simulink library "COMH"  (R2016b)
settings: Solver=ode45  StartTime=0.0  StopTime=10.0  RelTol=1e-3  EnableMultiTasking=on
undefined symbols (not defined in the file): CAL_EncoderSampleTime, CAL_FilterResetThd, CAL_fullCircle_DEG, CAL_MeasureNoise, CAL_NORTH, CAL_ProcessNoise, CAL_ROB_ERRVAL, CAL_ROBO_LENG_mm, CAL_thetaGain, CONST_ONE_UINT16, CONST_ZERO_UINT16, CONST_ZeroDeg, ENU_ROB_NONE
libraries: ThetaOverFlowFilter x1, movingAverage_1ms_to_5ms x1
settings Model: Creator=oelkawok  LastModifiedBy=oelkawok
settings DataIOCC: LimitDataPoints=on
settings OptimizationCC: LifeSpan=inf
settings DebuggingCC: AllowSymbolicDim=off  SFUnexpectedBacktrackingDiag=warning  SFNoUnconditionalDefaultTransitionDiag=warning  SFExecutionAtInitializationDiag=none
settings GRTTargetCC: TargetLangStandard=C89/C90 (ANSI)  GeneratePreprocessorConditionals=Disable all
settings ConfigComp: CovMetricSettings=dw  CovHtmlReporting=on  CovSaveCumulativeToWorkspaceVar=on  CovSaveSingleToWorkspaceVar=on  CovExternalEMLEnable=off

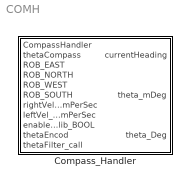
== system COMH ==
  Compass_Handler : Subsystem

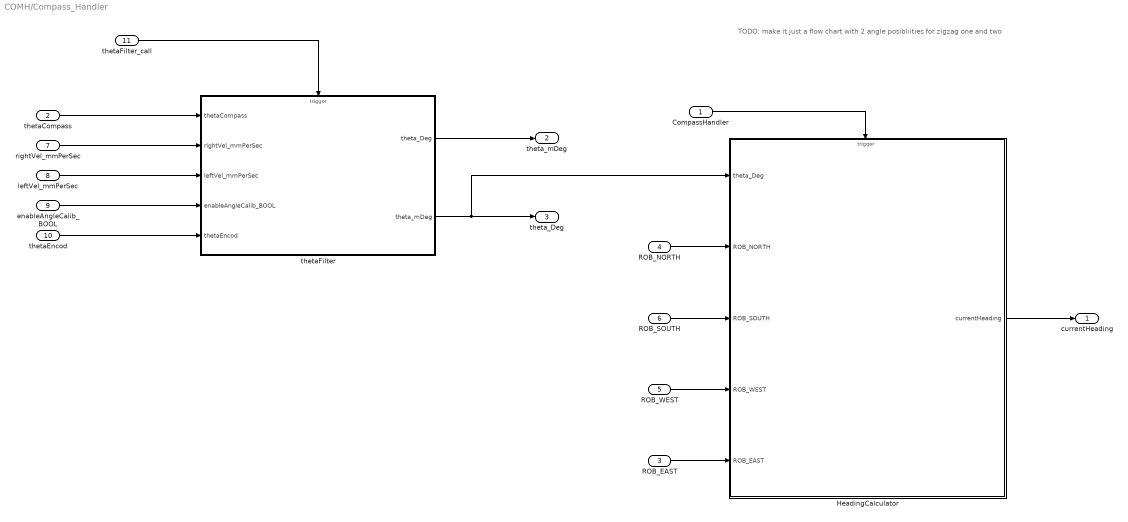
== system COMH/Compass_Handler ==
  note: TODO: make it just a flow chart with 2 angle posibliities for zigzag one and two
  CompassHandler : Inport  PortDimensions=1
  thetaCompass : Inport  Port=2
  ROB_EAST : Inport  Port=3  PortDimensions=1
  ROB_NORTH : Inport  Port=4  PortDimensions=1
  ROB_WEST : Inport  Port=5  PortDimensions=1
  ROB_SOUTH : Inport  Port=6  PortDimensions=1
  rightVel_mmPerSec : Inport  Port=7  PortDimensions=1
  leftVel_mmPerSec : Inport  Port=8  PortDimensions=1
  enableAngleCalib_BOOL : Inport  Port=9
  thetaEncod : Inport  Port=10  PortDimensions=1
  thetaFilter_call : Inport  Port=11  PortDimensions=1
  HeadingCalculator : Subsystem
      settings: RTWSystemCode=Nonreusable function  RTWFcnNameOpts=Use subsystem name  RTWFileNameOpts=Use subsystem name  FunctionInterfaceSpec=Allow arguments
  thetaFilter : Subsystem
      settings: RTWSystemCode=Nonreusable function  RTWFcnNameOpts=Use subsystem name  RTWFileNameOpts=Use subsystem name  FunctionInterfaceSpec=Allow arguments
  currentHeading : Outport
      settings: AttributesFormatString=|
      | Mode: %<OutputWhenDisabled>
      | Init: %<InitialOutput>
  theta_mDeg : Outport  Port=2
      settings: AttributesFormatString=|
      | Mode: %<OutputWhenDisabled>
      | Init: %<InitialOutput>
  theta_Deg : Outport  Port=3
      settings: AttributesFormatString=|
      | Mode: %<OutputWhenDisabled>
      | Init: %<InitialOutput>
  wires:
  CompassHandler/1 -> HeadingCalculator/Trigger
  HeadingCalculator/1(currentHeading) -> currentHeading/1
  ROB_EAST/1 -> HeadingCalculator/5(ROB_EAST)
  ROB_WEST/1 -> HeadingCalculator/4(ROB_WEST)
  ROB_SOUTH/1 -> HeadingCalculator/3(ROB_SOUTH)
  ROB_NORTH/1 -> HeadingCalculator/2(ROB_NORTH)
  thetaFilter/2(theta_mDeg) -> HeadingCalculator/1(theta_Deg), theta_Deg/1
  thetaCompass/1 -> thetaFilter/1(thetaCompass)
  rightVel_mmPerSec/1 -> thetaFilter/2(rightVel_mmPerSec)
  leftVel_mmPerSec/1 -> thetaFilter/3(leftVel_mmPerSec)
  enableAngleCalib_BOOL/1 -> thetaFilter/4(enableAngleCalib_BOOL)
  thetaEncod/1 -> thetaFilter/5(thetaEncod)
  thetaFilter/1(theta_Deg) -> theta_mDeg/1
  thetaFilter_call/1 -> thetaFilter/Trigger

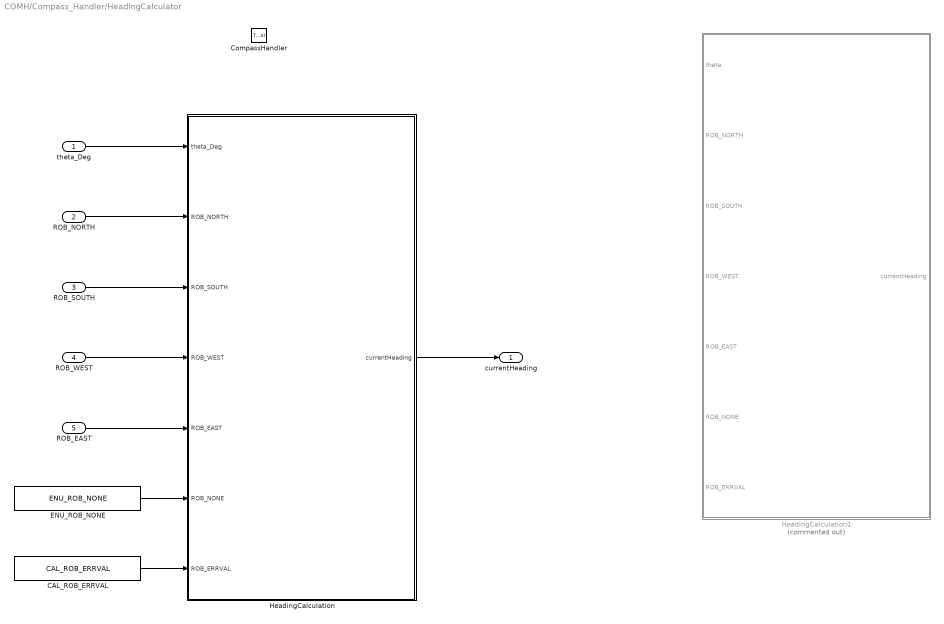
== system COMH/Compass_Handler/HeadingCalculator ==
  theta_Deg : Inport
  ROB_NORTH : Inport  Port=2  PortDimensions=1
  ROB_SOUTH : Inport  Port=3  PortDimensions=1
  ROB_WEST : Inport  Port=4  PortDimensions=1
  ROB_EAST : Inport  Port=5  PortDimensions=1
  CompassHandler : TriggerPort  TriggerType=function-call  VariantControl=Variant
      settings: AttributesFormatString=Mode: %<StatesWhenEnabling>
  CAL_ROB_ERRVAL : Constant  Value=CAL_ROB_ERRVAL
  ENU_ROB_NONE : Constant  Value=ENU_ROB_NONE
  HeadingCalculation : Stateflow chart  TreatAsAtomicUnit=on
  HeadingCalculation1 : Stateflow chart  Commented=on  TreatAsAtomicUnit=on
  currentHeading : Outport
      settings: AttributesFormatString=|
      | Mode: %<OutputWhenDisabled>
      | Init: %<InitialOutput>
  wires:
  theta_Deg/1 -> HeadingCalculation/1(theta_Deg)
  HeadingCalculation/1(currentHeading) -> currentHeading/1
  ROB_NORTH/1 -> HeadingCalculation/2(ROB_NORTH)
  ROB_SOUTH/1 -> HeadingCalculation/3(ROB_SOUTH)
  ROB_WEST/1 -> HeadingCalculation/4(ROB_WEST)
  ROB_EAST/1 -> HeadingCalculation/5(ROB_EAST)
  CAL_ROB_ERRVAL/1 -> HeadingCalculation/7(ROB_ERRVAL)
  ENU_ROB_NONE/1 -> HeadingCalculation/6(ROB_NONE)

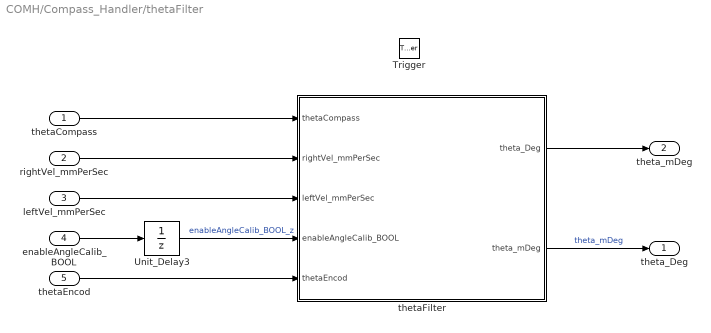
== system COMH/Compass_Handler/thetaFilter ==
  thetaCompass : Inport
  rightVel_mmPerSec : Inport  Port=2  PortDimensions=1
  leftVel_mmPerSec : Inport  Port=3  PortDimensions=1
  enableAngleCalib_BOOL : Inport  Port=4
  thetaEncod : Inport  Port=5  PortDimensions=1
  Trigger : TriggerPort  TriggerType=function-call  VariantControl=Variant  PortDimensions=1
  Unit_Delay3 : UnitDelay  SampleTime=-1
      settings: AttributesFormatString=Init: %<InitialCondition>
  thetaFilter : Subsystem
  theta_Deg : Outport
  theta_mDeg : Outport  Port=2
  wires:
  enableAngleCalib_BOOL/1 -> Unit_Delay3/1
  thetaFilter/1(theta_Deg) -> theta_mDeg/1
  thetaEncod/1 -> thetaFilter/5(thetaEncod)
  leftVel_mmPerSec/1 -> thetaFilter/3(leftVel_mmPerSec)
  thetaFilter/2(theta_mDeg) -> theta_Deg/1  "theta_mDeg"
  thetaCompass/1 -> thetaFilter/1(thetaCompass)
  Unit_Delay3/1 -> thetaFilter/4(enableAngleCalib_BOOL)  "enableAngleCalib_BOOL_z"
  rightVel_mmPerSec/1 -> thetaFilter/2(rightVel_mmPerSec)

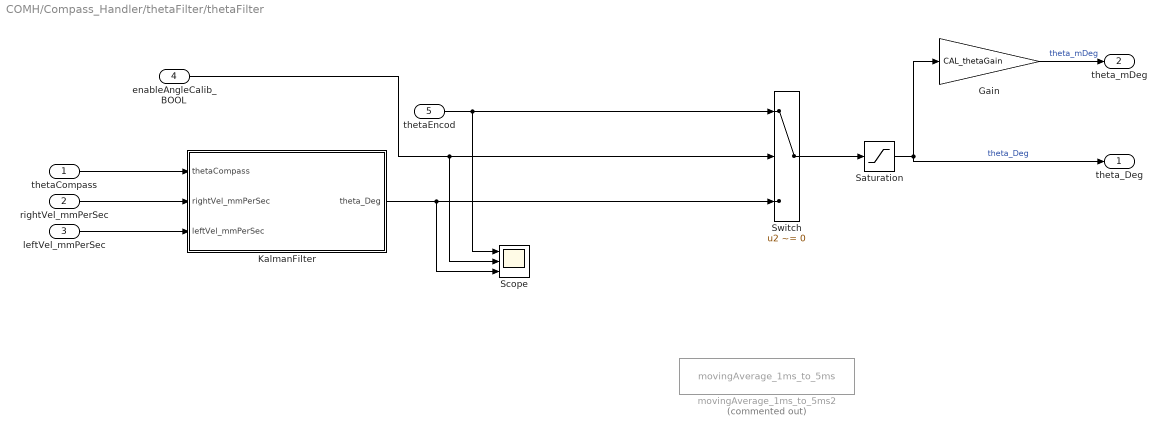
== system COMH/Compass_Handler/thetaFilter/thetaFilter ==
  thetaCompass : Inport
  rightVel_mmPerSec : Inport  Port=2  PortDimensions=1
  leftVel_mmPerSec : Inport  Port=3  PortDimensions=1
  enableAngleCalib_BOOL : Inport  Port=4
  thetaEncod : Inport  Port=5  PortDimensions=1
  Gain : Gain  Gain=CAL_thetaGain
  KalmanFilter : Subsystem
  Saturation : Saturate  UpperLimit=CAL_fullCircle_DEG  LowerLimit=CONST_ZERO_UINT16
      settings: AttributesFormatString=|
      | upper = %<UpperLimit>
      | lower = %<LowerLimit>
  Scope : Scope  NumInputPorts=3
  Switch : Switch  Criteria=u2 ~= 0
  movingAverage_1ms_to_5ms2 : movingAverage_1ms_to_5ms/movingAverage_1ms_to_5ms  Commented=on
  theta_Deg : Outport
  theta_mDeg : Outport  Port=2
  wires:
  KalmanFilter/1(theta_Deg) -> Scope/3, Switch/3
  thetaEncod/1 -> Scope/1, Switch/1
  Gain/1 -> theta_mDeg/1  "theta_mDeg"
  Saturation/1 -> Gain/1, theta_Deg/1  "theta_Deg"
  enableAngleCalib_BOOL/1 -> Switch/2, Scope/2
  Switch/1 -> Saturation/1
  thetaCompass/1 -> KalmanFilter/1(thetaCompass)
  leftVel_mmPerSec/1 -> KalmanFilter/3(leftVel_mmPerSec)
  rightVel_mmPerSec/1 -> KalmanFilter/2(rightVel_mmPerSec)

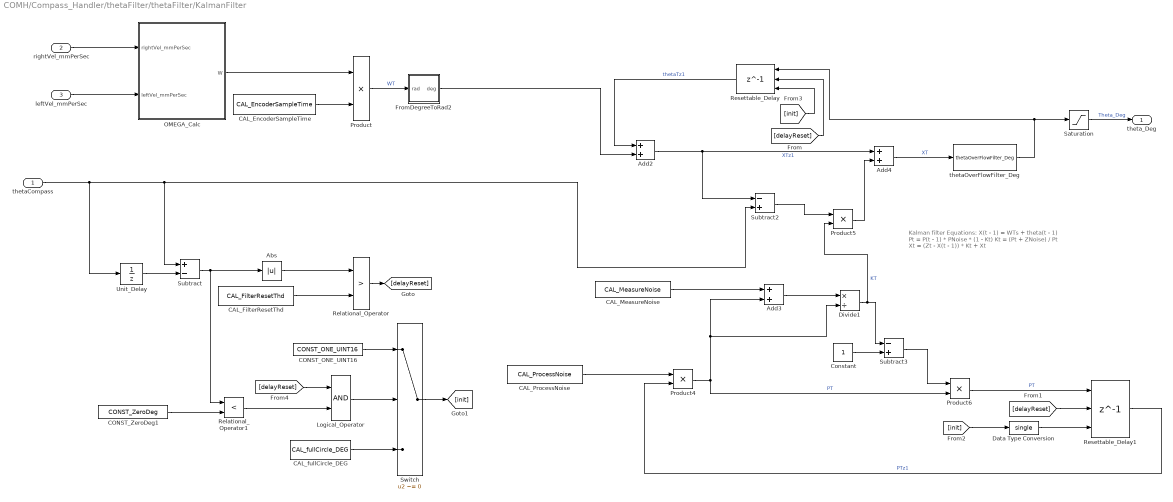
== system COMH/Compass_Handler/thetaFilter/thetaFilter/KalmanFilter ==
  note: Kalman filter Equations:
      | X(t - 1) = WTs + theta(t - 1)
      | Pt = P(t - 1) * PNoise * (1 - Kt)
      | Kt = (Pt + ZNoise) / Pt
      | Xt = (Zt - X(t - 1)) * Kt + Xt
  thetaCompass : Inport
  rightVel_mmPerSec : Inport  Port=2
  leftVel_mmPerSec : Inport  Port=3
  Abs : Abs  SaturateOnIntegerOverflow=on
  Add2 : Sum  OutDataTypeStr=Inherit: Same as first input
  Add3 : Sum
  Add4 : Sum  OutDataTypeStr=single
  CAL_EncoderSampleTime : Constant  Value=CAL_EncoderSampleTime
  CAL_FilterResetThd : Constant  Value=CAL_FilterResetThd
  CAL_MeasureNoise : Constant  Value=CAL_MeasureNoise
  CAL_ProcessNoise : Constant  Value=CAL_ProcessNoise
  CAL_fullCircle_DEG : Constant  Value=CAL_fullCircle_DEG
  CONST_ONE_UINT16 : Constant  Value=CONST_ONE_UINT16
  CONST_ZeroDeg1 : Constant  Value=CONST_ZeroDeg
  Constant : Constant  OutDataTypeStr=single
  Data Type Conversion : DataTypeConversion  OutDataTypeStr=single
  Divide1 : Product  Inputs=*/  OutDataTypeStr=Inherit: Inherit via back propagation
  FromDegreeToRad2 : Subsystem
  Logical_Operator : Logic  AllPortsSameDT=off  OutDataTypeStr=boolean
  OMEGA_Calc : Subsystem
  Product : Product
  Product4 : Product  OutDataTypeStr=Inherit: Inherit via back propagation
  Product5 : Product  OutDataTypeStr=single
  Product6 : Product  OutDataTypeStr=Inherit: Inherit via back propagation
  Relational_Operator : RelationalOperator  Operator=>  OutDataTypeStr=boolean  RndMeth=Nearest
  Relational_Operator1 : RelationalOperator  Operator=<  OutDataTypeStr=boolean  RndMeth=Simplest
  Resettable_Delay : Delay  DelayLength=1  InitialConditionSource=Input port  ExternalReset=Rising
      settings: AttributesFormatString=Init: %<InitialCondition>  InputPortMap=u0,r5,p4
  Resettable_Delay1 : Delay  DelayLength=1  InitialConditionSource=Input port  ExternalReset=Rising
      settings: AttributesFormatString=Init: %<InitialCondition>  InputPortMap=u0,r5,p4
  Saturation : Saturate  UpperLimit=360  LowerLimit=0
      settings: AttributesFormatString=|
      | upper = %<UpperLimit>
      | lower = %<LowerLimit>
  Subtract : Sum  Inputs=+-
  Subtract2 : Sum  Inputs=-+
  Subtract3 : Sum  Inputs=-+  OutDataTypeStr=Inherit: Inherit via back propagation
  Switch : Switch  Criteria=u2 ~= 0
  Unit_Delay : UnitDelay  InitialCondition=CAL_NORTH  SampleTime=-1
      settings: AttributesFormatString=Init: %<InitialCondition>
  thetaOverFlowFilter_Deg : ThetaOverFlowFilter/thetaOverFlowFilter_Deg
  theta_Deg : Outport
  wires:
  Data Type Conversion/1 -> Resettable_Delay1/3
  [init] -> Data Type Conversion/1
  leftVel_mmPerSec/1 -> OMEGA_Calc/2(leftVel_mmPerSec)
  rightVel_mmPerSec/1 -> OMEGA_Calc/1(rightVel_mmPerSec)
  CAL_EncoderSampleTime/1 -> Product/2
  OMEGA_Calc/1(W) -> Product/1
  thetaCompass/1 -> Subtract/1, Subtract2/2, Unit_Delay/1
  Product/1 -> FromDegreeToRad2/1(rad)  "WT"
  Resettable_Delay/1 -> Add2/1  "thetaTz1"
  CAL_ProcessNoise/1 -> Product4/1
  Resettable_Delay1/1 -> Product4/2  "PTz1"
  Product4/1 -> Product6/2, Add3/2, Divide1/2  "PT"
  CAL_MeasureNoise/1 -> Add3/1
  Add3/1 -> Divide1/1
  Divide1/1 -> Subtract3/1, Product5/2  "KT"
  Add2/1 -> Subtract2/1, Add4/1  "XTz1"
  Subtract2/1 -> Product5/1
  Constant/1 -> Subtract3/2
  Subtract3/1 -> Product6/1
  Product6/1 -> Resettable_Delay1/1  "PT"
  Product5/1 -> Add4/2
  Add4/1 -> thetaOverFlowFilter_Deg/1  "XT"
  Unit_Delay/1 -> Subtract/2
  Subtract/1 -> Relational_Operator1/1, Abs/1
  [delayReset] -> Resettable_Delay/2
  [delayReset] -> Resettable_Delay1/2
  Abs/1 -> Relational_Operator/1
  Relational_Operator/1 -> [delayReset]
  thetaOverFlowFilter_Deg/1 -> Resettable_Delay/1, Saturation/1
  Saturation/1 -> theta_Deg/1  "Theta_Deg"
  CONST_ONE_UINT16/1 -> Switch/1
  CAL_fullCircle_DEG/1 -> Switch/3
  Switch/1 -> [init]
  [init] -> Resettable_Delay/3
  Relational_Operator1/1 -> Logical_Operator/2
  [delayReset] -> Logical_Operator/1
  Logical_Operator/1 -> Switch/2
  CONST_ZeroDeg1/1 -> Relational_Operator1/2
  FromDegreeToRad2/1(deg) -> Add2/2
  CAL_FilterResetThd/1 -> Relational_Operator/2

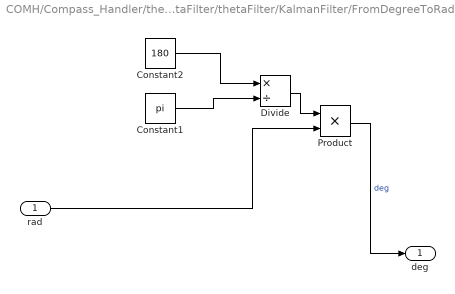
== system COMH/Compass_Handler/thetaFilter/thetaFilter/KalmanFilter/FromDegreeToRad2 ==
  rad : Inport
  Constant1 : Constant  Value=pi
  Constant2 : Constant  Value=180
  Divide : Product  Inputs=*/
  Product : Product
  deg : Outport
  wires:
  Divide/1 -> Product/1
  rad/1 -> Product/2
  Product/1 -> deg/1  "deg"
  Constant2/1 -> Divide/1
  Constant1/1 -> Divide/2

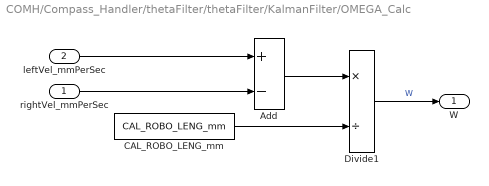
== system COMH/Compass_Handler/thetaFilter/thetaFilter/KalmanFilter/OMEGA_Calc ==
  rightVel_mmPerSec : Inport
  leftVel_mmPerSec : Inport  Port=2
  Add : Sum  Inputs=+-
  CAL_ROBO_LENG_mm : Constant  Value=CAL_ROBO_LENG_mm
  Divide1 : Product  Inputs=*/  OutDataTypeStr=single
  W : Outport
  wires:
  leftVel_mmPerSec/1 -> Add/1
  rightVel_mmPerSec/1 -> Add/2
  CAL_ROBO_LENG_mm/1 -> Divide1/2
  Divide1/1 -> W/1  "W"
  Add/1 -> Divide1/1

== stateflow chart COMH/Compass_Handler/HeadingCalculator/HeadingCalculation1 ==
  settings: description=Chart for calculation of heading. Could be used as state but not used
  state CalcHeadingEastZero
    (default) -> (junction 2)
    (junction 2) -> (junction 3) [order 1] : [(theta_OUT <= ROB_NORTH + ROB_ERRVAL) && (theta_OUT >= ROB_NORTH - ROB_ERRVAL)]//NORTH
    (junction 2) -> (junction 4) [order 2]
    (junction 3) -> (junction 17) : {currentHeading = ROB_NORTH;}
    (junction 4) -> (junction 5) [order 1] : [(theta_OUT <= ROB_SOUTH + ROB_ERRVAL) && (theta_OUT >= ROB_SOUTH - ROB_ERRVAL)]//SOUTH
    (junction 4) -> (junction 6) [order 2]
    (junction 5) -> (junction 16) : {currentHeading = ROB_SOUTH;}
    (junction 6) -> (junction 7) [order 1] : [(theta_OUT <= ROB_EAST + ROB_ERRVAL) || (theta_OUT >= CAL_fullCircle_DEG - ROB_ERRVAL)]//EAST
    (junction 6) -> (junction 8) [order 2]
    (junction 7) -> (junction 15) : {currentHeading = ROB_EAST;}
    (junction 8) -> (junction 9) [order 1] : [(theta_OUT <= ROB_WEST + ROB_ERRVAL) && (theta_OUT >= ROB_WEST - ROB_ERRVAL)]//WEST
    (junction 8) -> (junction 12) [order 2] : {currentHeading = ROB_NONE;}
    (junction 9) -> (junction 14) : {currentHeading = ROB_WEST;}
    (junction 14) -> (junction 12)
    (junction 15) -> (junction 14)
    (junction 16) -> (junction 15)
    (junction 17) -> (junction 16)
    (junction 12) -> (junction 18)
  state initializeDirection
    entry:
    offset = theta;
  state Calc
    entry:
    theta_OUT = theta;
    //remove for now - offset
  state CalcHeadingSouthZero
    (default) -> (junction 68)
    (junction 68) -> (junction 69) [order 1] : [(theta_OUT <= ROB_NORTH + ROB_ERRVAL) && (theta_OUT >= ROB_NORTH - ROB_ERRVAL)]//NORTH
    (junction 68) -> (junction 70) [order 2]
    (junction 69) -> (junction 80) : {currentHeading = ROB_NORTH;}
    (junction 70) -> (junction 71) [order 1] : [(theta_OUT <= ROB_SOUTH + ROB_ERRVAL) || (theta_OUT >= CAL_fullCircle_DEG - ROB_ERRVAL)]//SOUTH
    (junction 70) -> (junction 72) [order 2]
    (junction 71) -> (junction 79) : {currentHeading = ROB_SOUTH;}
    (junction 72) -> (junction 73) [order 1] : [(theta_OUT <= ROB_EAST + ROB_ERRVAL) && (theta_OUT >= ROB_EAST - ROB_ERRVAL)]//EAST
    (junction 72) -> (junction 74) [order 2]
    (junction 73) -> (junction 78) : {currentHeading = ROB_EAST;}
    (junction 74) -> (junction 75) [order 1] : [(theta_OUT <= ROB_WEST + ROB_ERRVAL) && (theta_OUT >= ROB_WEST - ROB_ERRVAL)]//WEST
    (junction 74) -> (junction 76) [order 2] : {currentHeading = ROB_NONE;}
    (junction 75) -> (junction 77) : {currentHeading = ROB_WEST;}
    (junction 77) -> (junction 76)
    (junction 78) -> (junction 77)
    (junction 79) -> (junction 78)
    (junction 80) -> (junction 79)
    (junction 76) -> (junction 81)
  CalcHeadingEastZero -> (junction 64) : /theta_OUT = theta;
  (junction 64) -> CalcHeadingEastZero [order 1] : [ROB_EAST == 0]
  Calc -> (junction 64) [order 2] : [hasChanged(theta)]
  CalcHeadingSouthZero -> (junction 64) : /theta_OUT = theta;
  (junction 64) -> CalcHeadingSouthZero [order 2] : [ROB_SOUTH == 0]
  Calc -> (junction 64) [order 3] : [theta_OUT < 0]
      | /
      | theta_OUT := theta_OUT + CAL_fullCircle_DEG;
  (junction 57) -> (junction 64) : /theta_OUT = ROB_ERRVAL;
  (junction 64) -> Calc [order 3]
  (default) -> initializeDirection
  initializeDirection -> Calc
  Calc -> (junction 57) [order 1] : [theta_OUT < ROB_ERRVAL]
  data: theta input; ROB_NORTH input; ROB_SOUTH input; ROB_WEST input; ROB_EAST input; ROB_NONE input; ROB_ERRVAL input; theta_OUT local int16; currentHeading output uint16; offset local int16; CAL_fullCircle_DEG constant uint16 =CAL_fullCircle_DEG

== stateflow chart COMH/Compass_Handler/HeadingCalculator/HeadingCalculation ==
  settings: description=Chart for calculation of heading. Could be used as state but not used
  state rangeFlg = thdOverflowRangeFlg(direction, theta) [function]
    (default) -> (junction 190)
    (junction 190) -> (junction 188) [order 1] : [direction - ROB_ERRVAL < 0]
    (junction 190) -> (junction 204) [order 2] : {
        | thdLower = direction - ROB_ERRVAL;
        | }
    (junction 188) -> (junction 182) : {
        | thdUpper = direction +  ROB_ERRVAL;
        | thdLower = (direction - ROB_ERRVAL) + CAL_fullCircle_DEG;
        | }
    (junction 204) -> (junction 199) [order 1] : [(direction +  ROB_ERRVAL) > CAL_fullCircle_DEG]
    (junction 204) -> (junction 202) [order 2] : {
        | thdUpper = direction +  ROB_ERRVAL;
        | }
    (junction 199) -> (junction 205) : {
        | thdUpper = (direction +  ROB_ERRVAL) - CAL_fullCircle_DEG;
        | thdLower = direction - ROB_ERRVAL;
        | }
    (junction 205) -> (junction 182)
    (junction 182) -> (junction 207) [order 1] : [theta >= thdLower || theta <= thdUpper]
    (junction 182) -> (junction 210) [order 2] : {
        | rangeFlg = false;
        | }
    (junction 207) -> (junction 208) : {
        | rangeFlg = true;
        | }
    (junction 202) -> (junction 221) [order 1] : [theta >= thdLower && theta <= thdUpper]
    (junction 202) -> (junction 216) [order 2] : {
        | rangeFlg = false;
        | }
    (junction 221) -> (junction 220) : {
        | rangeFlg = true;
        | }
    (junction 208) -> (junction 210)
    (junction 220) -> (junction 216)
  (default) -> (junction 109)
  (junction 109) -> (junction 110) [order 1] : [thdOverflowRangeFlg(ROB_NORTH, theta_Deg)]
  (junction 109) -> (junction 103) [order 2]
  (junction 110) -> (junction 116) : {currentHeading = ROB_NORTH;}
  (junction 103) -> (junction 106) [order 1] : [thdOverflowRangeFlg(ROB_SOUTH, theta_Deg)]
  (junction 103) -> (junction 104) [order 2]
  (junction 106) -> (junction 119) : {currentHeading = ROB_SOUTH;}
  (junction 104) -> (junction 107) [order 1] : [thdOverflowRangeFlg(ROB_EAST, theta_Deg)]
  (junction 104) -> (junction 105) [order 2]
  (junction 107) -> (junction 115) : {currentHeading = ROB_EAST;}
  (junction 105) -> (junction 108) [order 1] : [thdOverflowRangeFlg(ROB_WEST, theta_Deg)]
  (junction 108) -> (junction 114) : {currentHeading = ROB_WEST;}
  (junction 105) -> (junction 113) [order 2] : {currentHeading = ROB_NONE;}
  (junction 115) -> (junction 114)
  (junction 114) -> (junction 113)
  (junction 119) -> (junction 115)
  (junction 116) -> (junction 119)
  (junction 113) -> (junction 117)
  data: direction function_input double; rangeFlg function_output double; theta function_input double; theta_Deg input; ROB_NORTH input; ROB_SOUTH input; ROB_WEST input; ROB_EAST input; ROB_NONE input; ROB_ERRVAL input; currentHeading output uint16; CAL_fullCircle_DEG constant uint16 =CAL_fullCircle_DEG; thdUpper local int16; thdLower local int16
